simulink model "StateSpaceOL"  (R2018b)
settings: Solver=VariableStepAuto  StartTime=0.0  StopTime=5  RelTol=1e-3
values from neighbouring files (symbols this model uses):
  A = [[0, -4.0456, 0, 0,       0, 0, 0, 0, 0, 0, 0, 0] ... (first row only)    [StateSpaceAUV.m]    (also in StateSpaceAUVFromTf.m = [[-0.8635,      -0.345,           0,           0,           )
  B = [[0.0202, 0,      0,      0,      0,      0] ... (first row only)    [StateSpaceAUV.m]    (also in StateSpaceAUVFromTf.m = [[0.0625,       0,       0,       0,       0,       0])
  C = [[1, 0, 0, 0, 0, 0, 0, 0, 0, 0, 0, 0] ... (first row only)    [StateSpaceAUV.m]    (also in StateSpaceAUVFromTf.m = [[0.07013,   0.04396,         0,         0,         0,      )
  D = [[0, 0, 0, 0, 0, 0] ... (first row only)    [StateSpaceAUV.m]    (also in StateSpaceAUVFromTf.m = [[0   0   0   0   0   0])
settings Model: Creator=olavoie  LastModifiedBy=olavoie

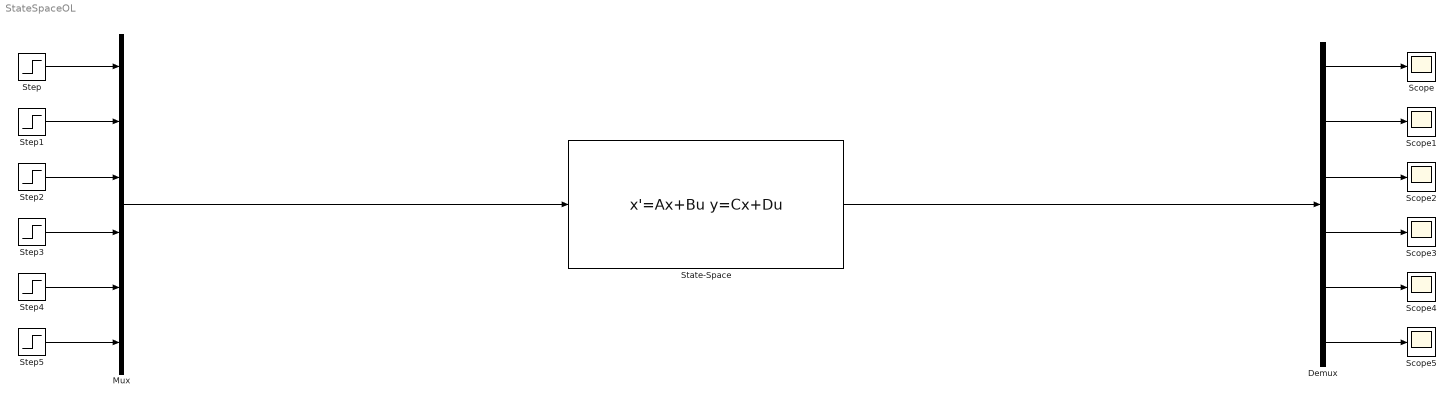
== system StateSpaceOL ==
  Demux : Demux  Outputs=6
  Mux : Mux  Inputs=6
  Scope{,1..5} (6 alike) : Scope
  State-Space : StateSpace  A=A  B=B  C=C  D=D  InitialCondition=0
  Step{,1..2,4} (4 alike) : Step  Time=0  After=30  SampleTime=0
  Step3 : Step  Time=0  After=0  SampleTime=0
  Step5 : Step  Time=0  SampleTime=0
  wires:
  Step2/1 -> Mux/3
  Step1/1 -> Mux/2
  Step/1 -> Mux/1
  Step3/1 -> Mux/4
  Step4/1 -> Mux/5
  Step5/1 -> Mux/6
  Demux/5 -> Scope4/1
  Demux/4 -> Scope3/1
  Demux/3 -> Scope2/1
  Demux/1 -> Scope/1
  Demux/2 -> Scope1/1
  Demux/6 -> Scope5/1
  Mux/1 -> State-Space/1
  State-Space/1 -> Demux/1
